simulink model "ros_simulation"  (R2019b)
settings: Solver=VariableStepAuto  StartTime=0.0  StopTime=120  RelTol=1e-3
undefined symbols (not defined in the file): eta_0, eta_ref, Orientation, Position, thrust_lower_limit, thrust_upper_limit
libraries: robotlib x2, robotcorelib x1, simulink x1
settings Model: Creator=loganfillo  LastModifiedBy=loganfillo
settings SolverCC: AlgebraicLoopSolver=LineSearch
settings OptimizationCC: UseDivisionForNetSlopeComputation=on

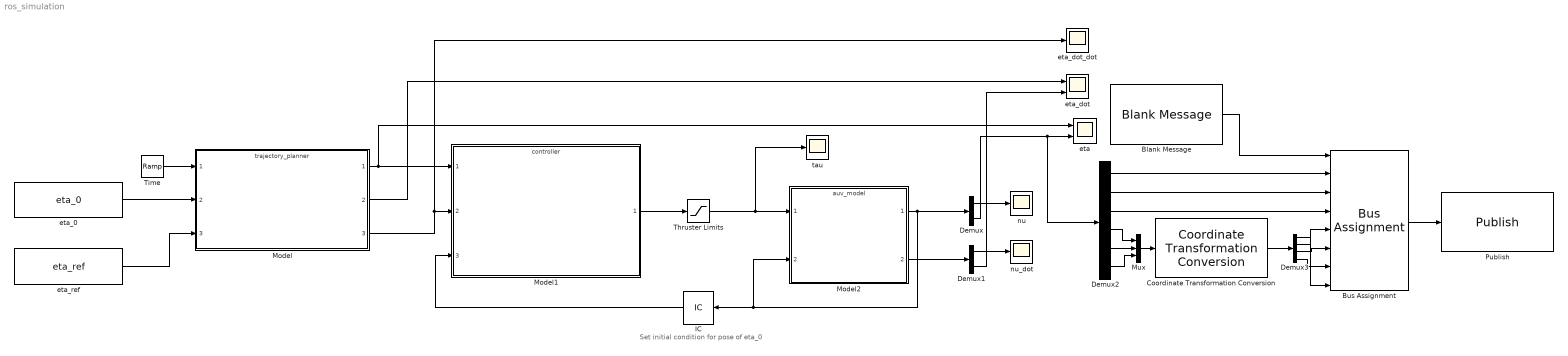
== system ros_simulation ==
  note: Set initial condition for pose of eta_0
  Blank Message : robotlib/Blank Message  messageClass=Message  entityType=geometry_msgs/Pose  messageType=geometry_msgs/Pose  SampleTime=inf
      settings: SourceProductName=ROS Toolbox
  Bus Assignment : BusAssignment  AssignedSignals=Position.X,Position.Y,Position.Z,Orientation.X,Orientation.Y,Orientation.Z,Orientation.W
  Coordinate Transformation Conversion : robotcorelib/Coordinate Transformation Conversion  InputRepresentation=Euler Angles  InputEulerSequence=XYZ  ShowTrVecInputPort=off  OutputRepresentation=Quaternion  OutputEulerSequence=ZYX  ShowTrVecOutputPort=on  SimulateUsing=Interpreted execution
      settings: SourceProductBaseCode=RO
  Demux : Demux  Outputs=[6,6]
  Demux1 : Demux  Outputs=[6,6]
  Demux2 : Demux  Outputs=6
  Demux3 : Demux
  IC : InitialCondition  Value=[0;0;0;0;0;0;eta_0]
  Model : ModelReference  ModelNameDialog=trajectory_planner.slx  SimulationMode=Normal  ModelReferenceVersion=1.30
  Model1 : ModelReference  ModelNameDialog=controller.slx  SimulationMode=Normal  ModelReferenceVersion=1.73
  Model2 : ModelReference  ModelNameDialog=auv_model  SimulationMode=Normal  ModelReferenceVersion=1.19
  Mux : Mux  Inputs=3
  Publish : robotlib/Publish  topicSource=Select from ROS network  topic=/g500/pose  messageType=geometry_msgs/Pose  messageQueueLength=1
      settings: SourceProductName=ROS Toolbox
  Thruster Limits : Saturate  UpperLimit=thrust_upper_limit  LowerLimit=thrust_lower_limit
  "Time " : simulink/Sources/Ramp  slope=1  start=0  InitialOutput=0
  eta : Scope  NumInputPorts=2
  eta_0 : Constant  Value=eta_0
  eta_dot : Scope  NumInputPorts=2
  eta_dot_dot : Scope
  eta_ref : Constant  Value=eta_ref
  nu : Scope
  nu_dot : Scope
  "tau " : Scope
  wires:
  Model1/1 -> Thruster Limits/1
  Model/3 -> eta_dot_dot/1, Model1/2
  Model2/1 -> Demux/1, Model2/2, IC/1
  "Time "/1 -> Model/1
  Demux1/2 -> eta_dot/2
  Demux1/1 -> nu_dot/1
  Model/2 -> eta_dot/1
  Model/1 -> Model1/1, eta/1
  Demux/1 -> nu/1
  Model2/2 -> Demux1/1
  Blank Message/1 -> Bus Assignment/1
  Bus Assignment/1 -> Publish/1
  Demux2/2 -> Bus Assignment/3
  Demux2/1 -> Bus Assignment/2
  Demux2/3 -> Bus Assignment/4
  Coordinate Transformation Conversion/1 -> Demux3/1
  Mux/1 -> Coordinate Transformation Conversion/1
  Demux2/4 -> Mux/1
  Demux2/5 -> Mux/2
  Demux2/6 -> Mux/3
  Demux3/1 -> Bus Assignment/8
  Demux3/2 -> Bus Assignment/5
  Demux3/3 -> Bus Assignment/6
  Demux3/4 -> Bus Assignment/7
  Thruster Limits/1 -> "tau "/1, Model2/1
  eta_ref/1 -> Model/3
  eta_0/1 -> Model/2
  Demux/2 -> Demux2/1, eta/2
  IC/1 -> Model1/3
